simulink model "AllModeswithRA"  (R2022a)
settings: Solver=FixedStepAuto  StartTime=0.0  StopTime=10.0  FixedStep=1e-3  RelTol=1e-3  EnableMultiTasking=on
undefined symbols (not defined in the file): D0, D1, D10, D11, D12, D13, D2, D3, D4, D5, D6, D7, D8, D9, PTA0, PTA1, PTA2, PTB23, PTB9, PTC16, PTC17, PTC2, PTC3, PTC4, PTD0, PTD1, PTD2, PTD3
libraries: frdmk64flib x15, dspstat3 x1
settings Model: ExtModeTrigDuration=5  Creator=kemij  LastModifiedBy=kemij
settings OptimizationCC: EnhancedBackFolding=on  PassReuseOutputArgsAs=Individual arguments  ZeroExternalMemoryAtStartup=off  ZeroInternalMemoryAtStartup=off  MaxStackSize=64  OptimizeBlockOrder=speed  DifferentSizesBufferReuse=on  OptimizationCustomize=off  EfficientTunableParamExpr=on
settings DebuggingCC: ParameterTunabilityLossMsg=error
settings HardwareCC: ProdBitPerPointer=32  ProdBitPerSizeT=32  ProdBitPerPtrDiffT=32  ProdLargestAtomicInteger=Long  ProdLargestAtomicFloat=Double  ProdWordSize=32  ProdHWDeviceType=ARM Compatible->ARM Cortex
settings SFSimCC: MATLABDynamicMemAlloc=off
settings RTWCC: SystemTargetFile=ert.tlc  HardwareBoard=NXP FRDM-K64F  TLCOptions="-aInlineSetEventsForThisBaseRateFcn=TLC_FALSE -aSuppressMultiTaskScheduler=TLC_FALSE  -aRateBasedStepFcn=0"  TemplateMakefile=ert_default_tmf  Toolchain=GNU Tools for ARM Embedded Processors
settings CodeAppCC: ForceParamTrailComments=on  IgnoreCustomStorageClasses=off  OperatorAnnotations=on  SimulinkDataObjDesc=on  SFDataObjDesc=on  InsertBlockDesc=on
settings ERTTargetCC: ExtModeTransport=4  ExtModeMexFile=sendToCommService

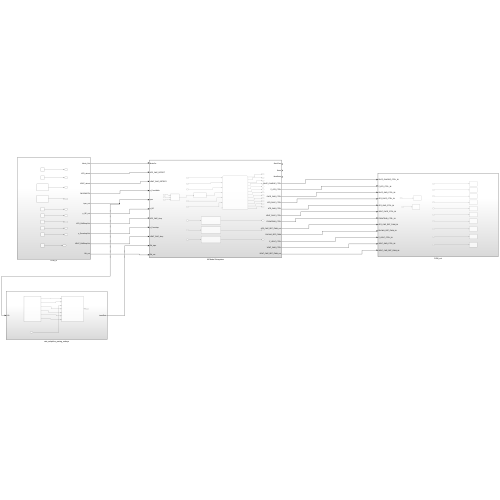
[thumbnail: Simulink's stored preview of the top-level diagram]
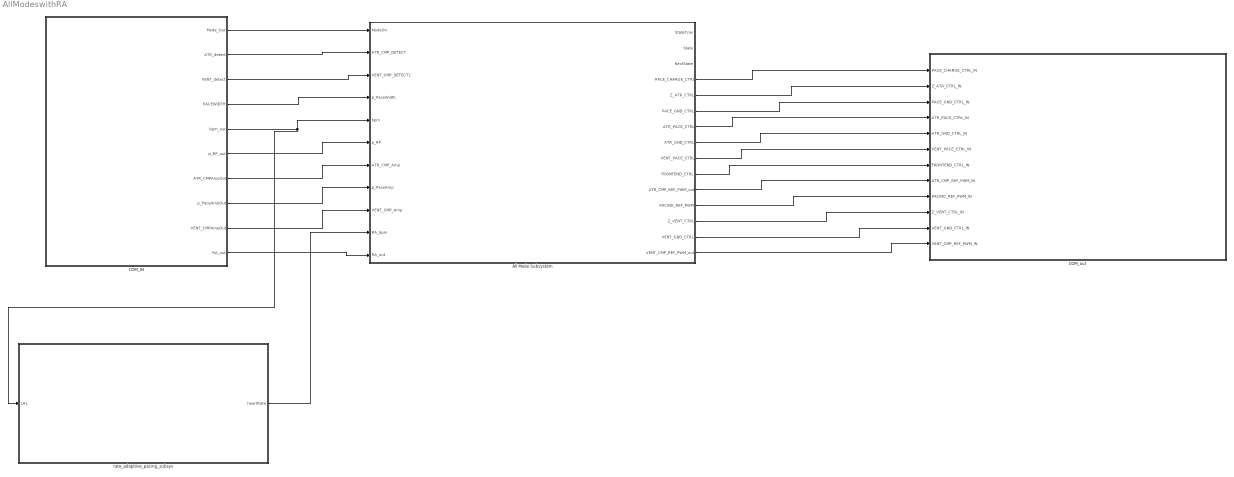
== system AllModeswithRA ==
  All Mode Subsystem : Subsystem
  COM_IN : Subsystem
  COM_out : Subsystem
  rate_adaptiive_pacing_subsys : Subsystem
  wires:
  COM_IN/3(VENT_detect) -> All Mode Subsystem/3(VENT_CMP_DETECT1)
  rate_adaptiive_pacing_subsys/1(heartRate) -> All Mode Subsystem/10(RA_bpm)
  COM_IN/10(RA_out) -> All Mode Subsystem/11(RA_out)
  COM_IN/2(ATR_detect) -> All Mode Subsystem/2(ATR_CMP_DETECT)
  All Mode Subsystem/13(Z_VENT_CTRL) -> COM_out/10(Z_VENT_CTRL_IN)
  All Mode Subsystem/15(VENT_CMP_REF_PWM_out) -> COM_out/12(VENT_CMP_REF_PWM_IN)
  COM_IN/6(p_RP_out) -> All Mode Subsystem/6(p_RP)
  COM_IN/1(Mode_Out) -> All Mode Subsystem/1(ModeOn)
  All Mode Subsystem/8(ATR_GND_CTRL) -> COM_out/5(ATR_GND_CTRL_IN)
  All Mode Subsystem/14(VENT_GND_CTRL) -> COM_out/11(VENT_GND_CTRL_IN)
  All Mode Subsystem/9(VENT_PACE_CTRL) -> COM_out/6(VENT_PACE_CTRL_IN)
  All Mode Subsystem/10(FRONTEND_CTRL) -> COM_out/7(FRONTEND_CTRL_IN)
  All Mode Subsystem/6(PACE_GND_CTRL) -> COM_out/3(PACE_GND_CTRL_IN)
  All Mode Subsystem/4(PACE_CHARGE_CTRL) -> COM_out/1(PACE_CHARGE_CTRL_IN)
  All Mode Subsystem/11(ATR_CMP_REF_PWM_out) -> COM_out/8(ATR_CMP_REF_PWM_IN)
  All Mode Subsystem/7(ATR_PACE_CTRL) -> COM_out/4(ATR_PACE_CTRL_IN)
  All Mode Subsystem/5(Z_ATR_CTRL) -> COM_out/2(Z_ATR_CTRL_IN)
  All Mode Subsystem/12(PACING_REF_PWM) -> COM_out/9(PACING_REF_PWM_IN)
  COM_IN/4(PACEWIDTH) -> All Mode Subsystem/4(p_PaceWidth)
  COM_IN/9(VENT_CMPAmpOut) -> All Mode Subsystem/9(VENT_CMP_Amp)
  COM_IN/5(bpm_out) -> rate_adaptiive_pacing_subsys/1(LRL), All Mode Subsystem/5(bpm)
  COM_IN/8(p_PaceAmpOut) -> All Mode Subsystem/8(p_PaceAmp)
  COM_IN/7(ATR_CMPAmpOut) -> All Mode Subsystem/7(ATR_CMP_Amp)

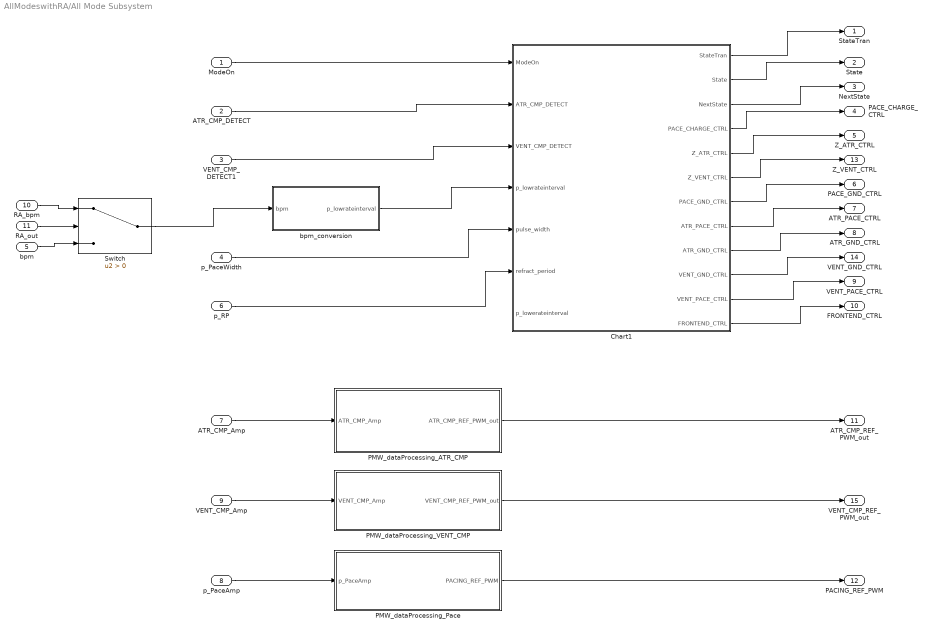
== system AllModeswithRA/All Mode Subsystem ==
  ModeOn : Inport
  ATR_CMP_DETECT : Inport  Port=2
  VENT_CMP_DETECT1 : Inport  Port=3
  p_PaceWidth : Inport  Port=4
  bpm : Inport  Port=5
  p_RP : Inport  Port=6
  ATR_CMP_Amp : Inport  Port=7
  p_PaceAmp : Inport  Port=8
  VENT_CMP_Amp : Inport  Port=9
  RA_bpm : Inport  Port=10
  RA_out : Inport  Port=11
  Chart1 : Stateflow chart  TreatAsAtomicUnit=on
      settings: PortSchema="{\"entries\":[{\"content\":{\"sides\":[{\"content\":{\"connectorIds\":[\"In1\",\"In2\",\"In3\",\"In4\",\"In5\",\"In6\",\"In7\"]},\"type\":\"ConnectorPlacement.EquallySpacedRectSide\",\"uuid\":\"7ea964f2-2529-4e69-b20d-c2fa6008c3a7\"},{\"content\":{\"connectorIds\":[\"Out12\",\"Out1\",\"Out11\",\"Out2\",\"Out3\",\"Out4\",\"Out5\",\"Out6\",\"Out7\",\"Out8\",\"Out9\",\"Out10\"],\"side\":\"RIGHT\"},\"type\":\"ConnectorPlacement.EquallySpacedRectSide\",\"uuid\":\"c561387b-bc02-43ab-893b-c9cb757a1c6a\"},{\"content\":{\"connectorIds\":[],\"side\":\"TOP\"},\"type\":\"ConnectorPlacement.EquallySpacedRectSide\",\"uuid\":\"1f667392-9a0f-4cad-82e3-6fe4d50b6af4\"}]},\"type\":\"ConnectorPlacement.EquallySpacedConnector\",\"uuid\":\"bd362c40-ffc0-452d-8626-3f1602423ca2\"}],\"packageUris\":[\"http://schema.mathworks.com/mf0/Connector/R2020b\"],\"version\":\"1.0\"}"
  PMW_dataProcessing_ATR_CMP : Subsystem
  PMW_dataProcessing_Pace : Subsystem
  PMW_dataProcessing_VENT_CMP : Subsystem
  Switch : Switch  Criteria=u2 > Threshold  SaturateOnIntegerOverflow=off  InputSameDT=off
  bpm_conversion : Subsystem
  StateTran : Outport
  State : Outport  Port=2
  NextState : Outport  Port=3
  PACE_CHARGE_CTRL : Outport  Port=4
  Z_ATR_CTRL : Outport  Port=5
  PACE_GND_CTRL : Outport  Port=6
  ATR_PACE_CTRL : Outport  Port=7
  ATR_GND_CTRL : Outport  Port=8
  VENT_PACE_CTRL : Outport  Port=9
  FRONTEND_CTRL : Outport  Port=10
  ATR_CMP_REF_PWM_out : Outport  Port=11
  PACING_REF_PWM : Outport  Port=12
  Z_VENT_CTRL : Outport  Port=13
  VENT_GND_CTRL : Outport  Port=14
  VENT_CMP_REF_PWM_out : Outport  Port=15
  wires:
  Chart1/10(FRONTEND_CTRL) -> FRONTEND_CTRL/1
  Chart1/9(VENT_PACE_CTRL) -> VENT_PACE_CTRL/1
  Chart1/7(ATR_GND_CTRL) -> ATR_GND_CTRL/1
  Chart1/6(ATR_PACE_CTRL) -> ATR_PACE_CTRL/1
  Chart1/5(PACE_GND_CTRL) -> PACE_GND_CTRL/1
  Chart1/3(Z_ATR_CTRL) -> Z_ATR_CTRL/1
  Chart1/2(PACE_CHARGE_CTRL) -> PACE_CHARGE_CTRL/1
  p_RP/1 -> Chart1/6(refract_period)
  p_PaceWidth/1 -> Chart1/5(pulse_width)
  ATR_CMP_DETECT/1 -> Chart1/2(ATR_CMP_DETECT)
  Chart1/1(State) -> State/1
  ModeOn/1 -> Chart1/1(ModeOn)
  Chart1/4(Z_VENT_CTRL) -> Z_VENT_CTRL/1
  Chart1/8(VENT_GND_CTRL) -> VENT_GND_CTRL/1
  VENT_CMP_DETECT1/1 -> Chart1/3(VENT_CMP_DETECT)
  ATR_CMP_Amp/1 -> PMW_dataProcessing_ATR_CMP/1(ATR_CMP_Amp)
  p_PaceAmp/1 -> PMW_dataProcessing_Pace/1(p_PaceAmp)
  VENT_CMP_Amp/1 -> PMW_dataProcessing_VENT_CMP/1(VENT_CMP_Amp)
  PMW_dataProcessing_Pace/1(PACING_REF_PWM) -> PACING_REF_PWM/1
  PMW_dataProcessing_VENT_CMP/1(VENT_CMP_REF_PWM_out) -> VENT_CMP_REF_PWM_out/1
  PMW_dataProcessing_ATR_CMP/1(ATR_CMP_REF_PWM_out) -> ATR_CMP_REF_PWM_out/1
  bpm_conversion/1(p_lowrateinterval) -> Chart1/4(p_lowrateinterval)
  Chart1/11(NextState) -> NextState/1
  Chart1/12(StateTran) -> StateTran/1
  RA_out/1 -> Switch/2
  RA_bpm/1 -> Switch/1
  bpm/1 -> Switch/3
  Switch/1 -> bpm_conversion/1(bpm)

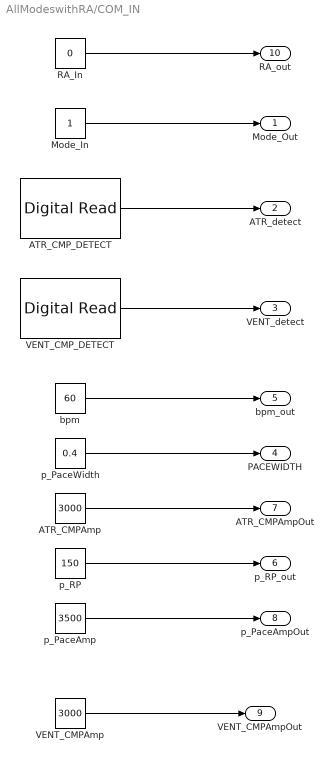
== system AllModeswithRA/COM_IN ==
  ATR_CMPAmp : Constant  Value=3000
  ATR_CMP_DETECT : frdmk64flib/Digital Read  Whichpin=PTC16 (D0)  SampleTime=-1
  Mode_In : Constant
  RA_In : Constant  Value=0
  VENT_CMPAmp : Constant  Value=3000
  VENT_CMP_DETECT : frdmk64flib/Digital Read  Whichpin=PTC17 (D1)  SampleTime=-1
  bpm : Constant  Value=60
  p_PaceAmp : Constant  Value=3500
  p_PaceWidth : Constant  Value=0.4
  p_RP : Constant  Value=150
  Mode_Out : Outport
  ATR_detect : Outport  Port=2
  VENT_detect : Outport  Port=3
  PACEWIDTH : Outport  Port=4
  bpm_out : Outport  Port=5
  p_RP_out : Outport  Port=6
  ATR_CMPAmpOut : Outport  Port=7
  p_PaceAmpOut : Outport  Port=8
  VENT_CMPAmpOut : Outport  Port=9
  RA_out : Outport  Port=10
  wires:
  Mode_In/1 -> Mode_Out/1
  ATR_CMP_DETECT/1 -> ATR_detect/1
  bpm/1 -> bpm_out/1
  ATR_CMPAmp/1 -> ATR_CMPAmpOut/1
  VENT_CMP_DETECT/1 -> VENT_detect/1
  p_PaceWidth/1 -> PACEWIDTH/1
  p_RP/1 -> p_RP_out/1
  p_PaceAmp/1 -> p_PaceAmpOut/1
  VENT_CMPAmp/1 -> VENT_CMPAmpOut/1
  RA_In/1 -> RA_out/1

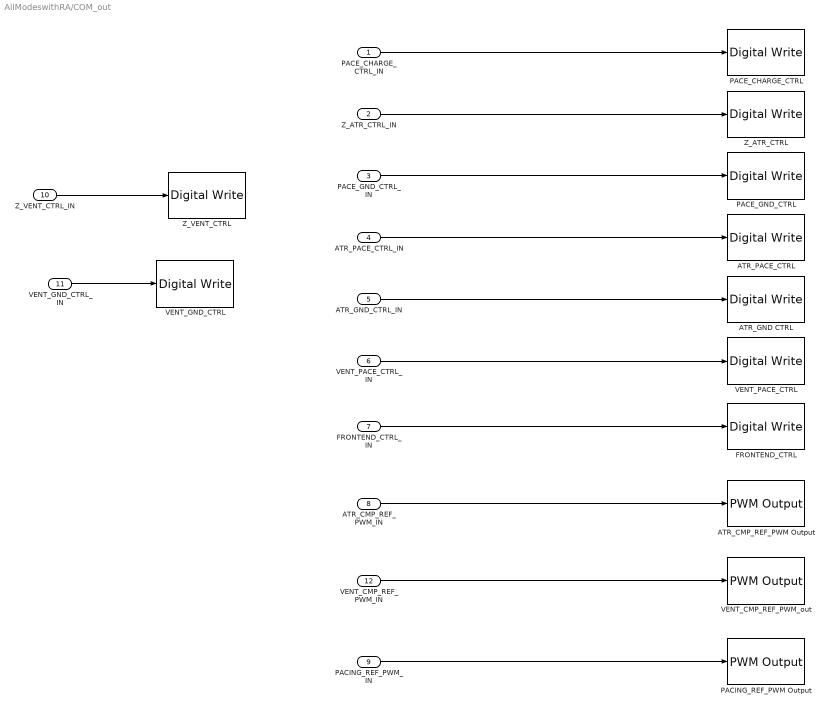
== system AllModeswithRA/COM_out ==
  PACE_CHARGE_CTRL_IN : Inport
  Z_ATR_CTRL_IN : Inport  Port=2
  PACE_GND_CTRL_IN : Inport  Port=3
  ATR_PACE_CTRL_IN : Inport  Port=4
  ATR_GND_CTRL_IN : Inport  Port=5
  VENT_PACE_CTRL_IN : Inport  Port=6
  FRONTEND_CTRL_IN : Inport  Port=7
  ATR_CMP_REF_PWM_IN : Inport  Port=8
  PACING_REF_PWM_IN : Inport  Port=9
  Z_VENT_CTRL_IN : Inport  Port=10
  VENT_GND_CTRL_IN : Inport  Port=11
  VENT_CMP_REF_PWM_IN : Inport  Port=12
  ATR_CMP_REF_PWM Output : frdmk64flib/PWM Output  Whichpin=PTC2 (D6)  InitialFrequency=2000  InitialDutyCycle=0
  ATR_GND CTRL : frdmk64flib/Digital Write  Whichpin=PTD2 (D11)
  ATR_PACE_CTRL : frdmk64flib/Digital Write  Whichpin=PTA0 (D8)
  FRONTEND_CTRL : frdmk64flib/Digital Write  Whichpin=PTD1 (D13)
  PACE_CHARGE_CTRL : frdmk64flib/Digital Write  Whichpin=PTB9 (D2)
  PACE_GND_CTRL : frdmk64flib/Digital Write  Whichpin=PTD0 (D10)
  PACING_REF_PWM Output : frdmk64flib/PWM Output  Whichpin=PTA2 (D5)  InitialFrequency=2000  InitialDutyCycle=0
  VENT_CMP_REF_PWM_out : frdmk64flib/PWM Output  Whichpin=PTA1 (D3)  InitialFrequency=2000  InitialDutyCycle=0
  VENT_GND_CTRL : frdmk64flib/Digital Write  Whichpin=PTD3 (D12)
  VENT_PACE_CTRL : frdmk64flib/Digital Write  Whichpin=PTC4 (D9)
  Z_ATR_CTRL : frdmk64flib/Digital Write  Whichpin=PTB23 (D4)
  Z_VENT_CTRL : frdmk64flib/Digital Write  Whichpin=PTC3 (D7)
  wires:
  PACE_CHARGE_CTRL_IN/1 -> PACE_CHARGE_CTRL/1
  PACE_GND_CTRL_IN/1 -> PACE_GND_CTRL/1
  Z_ATR_CTRL_IN/1 -> Z_ATR_CTRL/1
  ATR_PACE_CTRL_IN/1 -> ATR_PACE_CTRL/1
  ATR_GND_CTRL_IN/1 -> ATR_GND CTRL/1
  VENT_PACE_CTRL_IN/1 -> VENT_PACE_CTRL/1
  FRONTEND_CTRL_IN/1 -> FRONTEND_CTRL/1
  PACING_REF_PWM_IN/1 -> PACING_REF_PWM Output/1
  ATR_CMP_REF_PWM_IN/1 -> ATR_CMP_REF_PWM Output/1
  VENT_GND_CTRL_IN/1 -> VENT_GND_CTRL/1
  Z_VENT_CTRL_IN/1 -> Z_VENT_CTRL/1
  VENT_CMP_REF_PWM_IN/1 -> VENT_CMP_REF_PWM_out/1

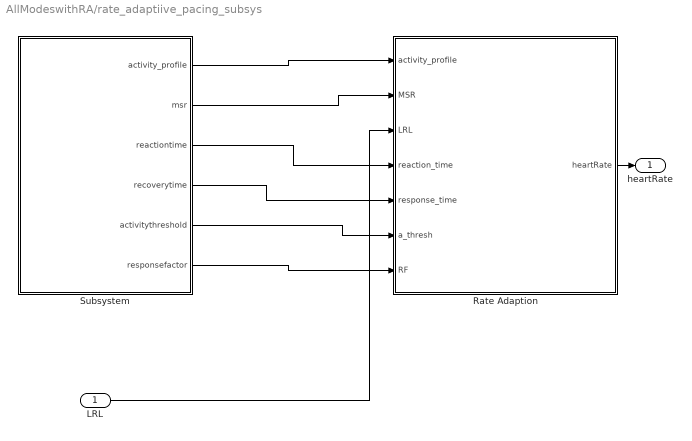
== system AllModeswithRA/rate_adaptiive_pacing_subsys ==
  LRL : Inport
  Rate Adaption : Subsystem
  Subsystem : Subsystem
  heartRate : Outport
  wires:
  Rate Adaption/1(heartRate) -> heartRate/1
  Subsystem/1(activity_profile) -> Rate Adaption/1(activity_profile)
  Subsystem/3(reactiontime) -> Rate Adaption/4(reaction_time)
  Subsystem/4(recoverytime) -> Rate Adaption/5(response_time)
  Subsystem/5(activitythreshold) -> Rate Adaption/6(a_thresh)
  Subsystem/6(responsefactor) -> Rate Adaption/7(RF)
  Subsystem/2(msr) -> Rate Adaption/2(MSR)
  LRL/1 -> Rate Adaption/3(LRL)

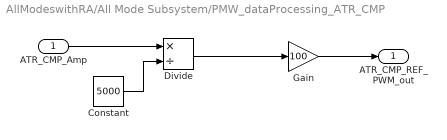
== system AllModeswithRA/All Mode Subsystem/PMW_dataProcessing_ATR_CMP ==
  ATR_CMP_Amp : Inport
  Constant : Constant  Value=5000
  Divide : Product  Inputs=*/
  Gain : Gain  Gain=100
  ATR_CMP_REF_PWM_out : Outport
  wires:
  Divide/1 -> Gain/1
  Constant/1 -> Divide/2
  ATR_CMP_Amp/1 -> Divide/1
  Gain/1 -> ATR_CMP_REF_PWM_out/1

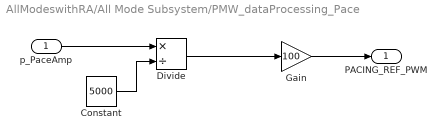
== system AllModeswithRA/All Mode Subsystem/PMW_dataProcessing_Pace ==
  p_PaceAmp : Inport
  Constant : Constant  Value=5000
  Divide : Product  Inputs=*/
  Gain : Gain  Gain=100
  PACING_REF_PWM : Outport
  wires:
  Divide/1 -> Gain/1
  Constant/1 -> Divide/2
  p_PaceAmp/1 -> Divide/1
  Gain/1 -> PACING_REF_PWM/1

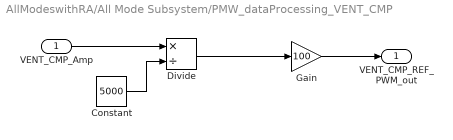
== system AllModeswithRA/All Mode Subsystem/PMW_dataProcessing_VENT_CMP ==
  VENT_CMP_Amp : Inport
  Constant : Constant  Value=5000
  Divide : Product  Inputs=*/
  Gain : Gain  Gain=100
  VENT_CMP_REF_PWM_out : Outport
  wires:
  Divide/1 -> Gain/1
  Constant/1 -> Divide/2
  VENT_CMP_Amp/1 -> Divide/1
  Gain/1 -> VENT_CMP_REF_PWM_out/1

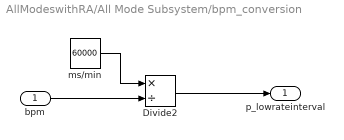
== system AllModeswithRA/All Mode Subsystem/bpm_conversion ==
  bpm : Inport
  Divide2 : Product  Inputs=*/
  ms/min : Constant  Value=60000
  p_lowrateinterval : Outport
  wires:
  ms/min/1 -> Divide2/1
  bpm/1 -> Divide2/2
  Divide2/1 -> p_lowrateinterval/1

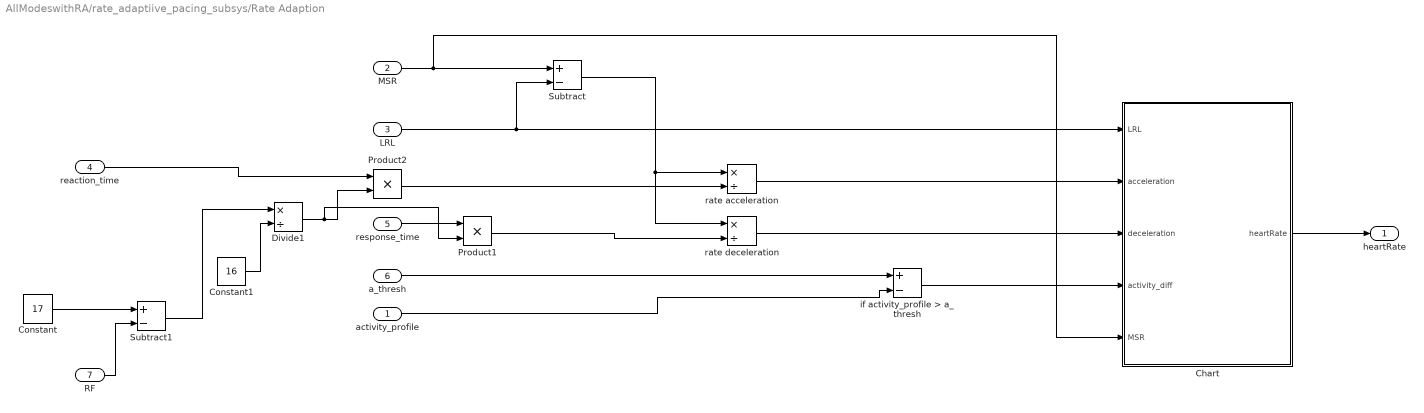
== system AllModeswithRA/rate_adaptiive_pacing_subsys/Rate Adaption ==
  activity_profile : Inport
  MSR : Inport  Port=2
  LRL : Inport  Port=3
  reaction_time : Inport  Port=4
  response_time : Inport  Port=5
  a_thresh : Inport  Port=6
  RF : Inport  Port=7
  Chart : Stateflow chart  TreatAsAtomicUnit=on
      settings: PortSchema="{\"entries\":[{\"content\":{\"sides\":[{\"content\":{\"connectorIds\":[\"In5\",\"In1\",\"In3\",\"In2\",\"In4\"]},\"type\":\"ConnectorPlacement.EquallySpacedRectSide\",\"uuid\":\"f1bfb65c-a3e0-488b-a51c-ed381b80a0d3\"},{\"content\":{\"connectorIds\":[\"Out1\"],\"side\":\"RIGHT\"},\"type\":\"ConnectorPlacement.EquallySpacedRectSide\",\"uuid\":\"38293472-2491-4ffe-ba83-6a5f72f7d4c8\"},{\"content\":{\"connectorIds\":[],\"side\":\"TOP\"},\"type\":\"ConnectorPlacement.EquallySpacedRectSide\",\"uuid\":\"d4d219f0-2dab-436b-b9c2-781e051d4797\"}]},\"type\":\"ConnectorPlacement.EquallySpacedConnector\",\"uuid\":\"faf9de58-f900-4f39-b014-8d2778c5d5cd\"}],\"packageUris\":[\"http://schema.mathworks.com/mf0/Connector/R2020b\"],\"version\":\"1.0\"}"
  Constant : Constant  Value=17
  Constant1 : Constant  Value=16
  Divide1 : Product  Inputs=*/
  Product1 : Product
  Product2 : Product
  Subtract : Sum  Inputs=+-
  Subtract1 : Sum  Inputs=+-
  if activity_profile > a_thresh : Sum  Inputs=+-
  rate acceleration : Product  Inputs=*/
  rate deceleration : Product  Inputs=*/
  heartRate : Outport
  wires:
  MSR/1 -> Chart/4(MSR), Subtract/1
  Chart/1(heartRate) -> heartRate/1
  LRL/1 -> Chart/5(LRL), Subtract/2
  Subtract/1 -> rate deceleration/1, rate acceleration/1
  RF/1 -> Subtract1/2
  rate acceleration/1 -> Chart/1(acceleration)
  rate deceleration/1 -> Chart/3(deceleration)
  if activity_profile > a_thresh/1 -> Chart/2(activity_diff)
  a_thresh/1 -> if activity_profile > a_thresh/1
  activity_profile/1 -> if activity_profile > a_thresh/2
  Product2/1 -> rate acceleration/2
  Constant/1 -> Subtract1/1
  Subtract1/1 -> Divide1/1
  Constant1/1 -> Divide1/2
  reaction_time/1 -> Product2/1
  Divide1/1 -> Product2/2, Product1/2
  response_time/1 -> Product1/1
  Product1/1 -> rate deceleration/2

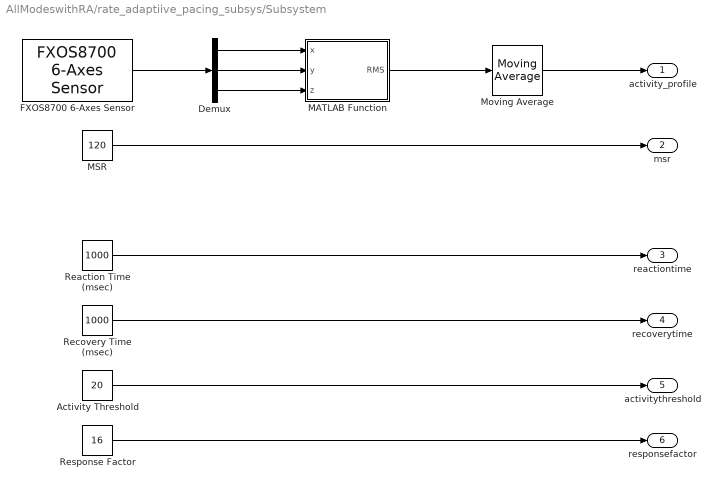
== system AllModeswithRA/rate_adaptiive_pacing_subsys/Subsystem ==
  Activity Threshold : Constant  Value=20
  Demux : Demux  Outputs=3
  FXOS8700 6-Axes Sensor : frdmk64flib/FXOS8700 6-Axes Sensor  Activesensor=Accelerometer only  ODR=800Hz  HybridODR=400Hz  Accelfullrange=-4g to +4g  SampleTime=-1
  MATLAB Function : MATLAB Function  TreatAsAtomicUnit=on
  MSR : Constant  Value=120
  Moving Average : dspstat3/Moving Average  Method=Sliding window  ForgettingFactorPort=off  SpecifyWindowLength=on  WindowLength=4  ForgettingFactor=0.9  SimulateUsing=Code generation
  Reaction Time (msec) : Constant  Value=1000
  Recovery Time (msec) : Constant  Value=1000
  Response Factor : Constant  Value=16
  activity_profile : Outport
  msr : Outport  Port=2
  reactiontime : Outport  Port=3
  recoverytime : Outport  Port=4
  activitythreshold : Outport  Port=5
  responsefactor : Outport  Port=6
  wires:
  Moving Average/1 -> activity_profile/1
  MSR/1 -> msr/1
  Reaction Time (msec)/1 -> reactiontime/1
  Recovery Time (msec)/1 -> recoverytime/1
  Activity Threshold/1 -> activitythreshold/1
  Response Factor/1 -> responsefactor/1
  Demux/3 -> MATLAB Function/3(z)
  Demux/2 -> MATLAB Function/2(y)
  MATLAB Function/1(RMS) -> Moving Average/1
  Demux/1 -> MATLAB Function/1(x)
  FXOS8700 6-Axes Sensor/1 -> Demux/1

== matlab function AllModeswithRA/rate_adaptiive_pacing_subsys/Subsystem/MATLAB Function ==
  data: x input; RMS output; y input; z input
function RMS = calc_RMS(x,y,z)

RMS = sqrt((x^2 + y^2 + z^2)/3.0);

== stateflow chart AllModeswithRA/All Mode Subsystem/Chart1 ==
  state AOO_Charging_Discharging
    entry:
    StateTran = false
    NextState = 0
    ATR_PACE_CTRL = false
    VENT_PACE_CTRL=false
    PACE_CHARGE_CTRL = true
    ATR_GND_CTRL = true
    PACE_GND_CTRL = true
    Z_ATR_CTRL=false
    State = 1
    exit:
    StateTran = true
  state AOO_Pace_Heart
    entry:
    StateTran = false
    NextState = 0
    ATR_PACE_CTRL = true
    PACE_CHARGE_CTRL = false
    PACE_GND_CTRL = true
    ATR_GND_CTRL = false
    State = 2
    exit:
    StateTran = true
  state VOO_VENT_Charging_Discharging
    entry:
    NextState = 0
    VENT_PACE_CTRL = false
    ATR_PACE_CTRL = false
    PACE_CHARGE_CTRL = true
    VENT_GND_CTRL = true
    PACE_GND_CTRL = true
    Z_VENT_CTRL=false
    State = 3
    StateTran = false
    exit:
    StateTran = true
  state VOO_VENT_Pace_Heart
    entry:
    NextState = 0
    StateTran = false
    VENT_PACE_CTRL = true
    PACE_CHARGE_CTRL = false
    PACE_GND_CTRL = true
    VENT_GND_CTRL = false
    State = 4
    exit:
    StateTran = true
  state AAI_Pulse_Sensed
    entry:
    NextState = 0
    %FRONTEND_CTRL=false
    State = 6
    StateTran = false
    exit:
    StateTran = true
    wait_time=refract_period
  state StateOff
    %This state tells the pacemaker which
    %mode it should run, which is decided
    %by ModeOn and is checked on the
    %transistion conditions.
    entry:
    %Initialize all states to 0 or false, since
    %the pacemaker should do nothing in this
    %state.
    StateTran = false
    State = 0
    NextState = 0
    PACE_CHARGE_CTRL = false
    Z_ATR_CTRL = false
    Z_VENT_CTRL = false
    PACE_GND_CTRL = false
    ATR_PACE_CTRL = false
    ATR_GND_CTRL = false
    VENT_GND_CTRL = false
    VENT_PACE_CTRL = false
    FRONTEND_CTRL = false
    exit:
    StateTran = true
    wait_time=pulse_width
  state AAI_Charging_Discharging
    entry:
    NextState = 0
    ATR_PACE_CTRL = false
    VENT_PACE_CTRL=false
    PACE_CHARGE_CTRL = true
    ATR_GND_CTRL = true
    PACE_GND_CTRL = true
    Z_ATR_CTRL=false
    FRONTEND_CTRL=true
    State = 5
    StateTran = false
    exit:
    StateTran = true
  state AAI_Pace_Heart
    entry:
    NextState = 0
    ATR_PACE_CTRL = true
    PACE_CHARGE_CTRL = false
    PACE_GND_CTRL = true
    ATR_GND_CTRL = false
    State = 7
    StateTran = false
    exit:
    StateTran = true
    wait_time=pulse_width
  state VVI_Pulse_Sensed
    entry:
    NextState = 0
    %FRONTEND_CTRL=false
    State = 9
    StateTran = false
    exit:
    StateTran = true
    wait_time=refract_period
  state VVI_Charging_Discharging
    entry:
    NextState = 0
    ATR_PACE_CTRL = false
    VENT_PACE_CTRL=false
    PACE_CHARGE_CTRL = true
    VENT_GND_CTRL = true
    PACE_GND_CTRL = true
    Z_VENT_CTRL=false
    FRONTEND_CTRL=true
    State = 8
    StateTran = false
    exit:
    StateTran = true
  state VVI_Pace_Heart
    entry:
    NextState = 0
    VENT_PACE_CTRL = true
    PACE_CHARGE_CTRL = false
    PACE_GND_CTRL = true
    VENT_GND_CTRL = false
    State = 10
    StateTran = false
    exit:
    StateTran = true
    wait_time=pulse_width
  AOO_Charging_Discharging -> AOO_Pace_Heart : after(p_lowrateinterval-pulse_width,msec) / {NextState = 2}
  StateOff -> AOO_Charging_Discharging [order 4] : [ModeOn==1] / {NextState = 1}
  AOO_Pace_Heart -> AOO_Charging_Discharging : after(pulse_width,msec) / {NextState = 1}
  VOO_VENT_Charging_Discharging -> VOO_VENT_Pace_Heart : after(p_lowerateinterval-pulse_width,msec) / {NextState = 4}
  VOO_VENT_Pace_Heart -> VOO_VENT_Charging_Discharging : after(pulse_width,msec) / {NextState = 3}
  StateOff -> VOO_VENT_Charging_Discharging [order 3] : [ModeOn==2] / {NextState = 3}
  (default) -> StateOff
  AAI_Pulse_Sensed -> AAI_Charging_Discharging : [after(refract_period,msec)] / {NextState = 5}
  AAI_Charging_Discharging -> AAI_Pulse_Sensed [order 2] : [ATR_CMP_DETECT == 1] / {NextState = 6}
  StateOff -> AAI_Charging_Discharging [order 1] : [ModeOn==3] / {NextState = 5}
  AAI_Charging_Discharging -> AAI_Pace_Heart [order 1] : [after(p_lowrateinterval-wait_time,msec)] / {NextState = 7}
  AAI_Pace_Heart -> AAI_Charging_Discharging : after(pulse_width,msec) / {NextState = 5}
  StateOff -> VVI_Charging_Discharging [order 2] : [ModeOn==4] / {NextState = 8}
  VVI_Pulse_Sensed -> VVI_Charging_Discharging : [after(refract_period,msec)] / {NextState = 8}
  VVI_Charging_Discharging -> VVI_Pulse_Sensed [order 2] : [VENT_CMP_DETECT == 1] / {NextState = 9}
  VVI_Charging_Discharging -> VVI_Pace_Heart [order 1] : [after(p_lowrateinterval-wait_time,msec)] / {NextState = 10}
  VVI_Pace_Heart -> VVI_Charging_Discharging : after(pulse_width,msec) / {NextState = 8}
  data: ModeOn input; State output int8; ATR_CMP_DETECT input boolean; VENT_CMP_DETECT input; p_lowrateinterval input; PACE_CHARGE_CTRL output boolean; Z_ATR_CTRL output boolean; Z_VENT_CTRL output boolean; PACE_GND_CTRL output boolean; ATR_PACE_CTRL output boolean; ATR_GND_CTRL output boolean; VENT_GND_CTRL output boolean; pulse_width input; VENT_PACE_CTRL output boolean; refract_period input; FRONTEND_CTRL output boolean; NextState output int8; StateTran output boolean; wait_time local; p_lowerateinterval input

== stateflow chart AllModeswithRA/rate_adaptiive_pacing_subsys/Rate Adaption/Chart ==
  state IncreaseHeartRate
    during:
    activity_time = elapsed(msec)
    heartRate = heartRate + acceleration*activity_time
  state HOLDSensorRate
    during:
    heartRate = MSR
  state IDLE
    entry:
    heartRate = LRL
    activity_time = 0
    zero_activity_time = 0
  state ActivitySensed
    %activity has been sensed
  state HOLDLRL
    during:
    heartRate = LRL
  state DecreaseHeartRate
    % decrease rate until there is zero activity (0 bpm)
    during:
    zero_activity_time = elapsed(msec)
    heartRate = heartRate - deceleration*zero_activity_time
  (junction 15) -> IncreaseHeartRate [order 1] : [heartRate + acceleration*activity_time <MSR]
  IncreaseHeartRate -> (junction 26) : [heartRate==MSR || activity_diff<=0 ]
  ActivitySensed -> (junction 15) [order 2] : [activity_diff > 0]
  (junction 15) -> HOLDSensorRate [order 2] : [heartRate + acceleration*activity_time >= MSR]
  HOLDSensorRate -> (junction 26) : [activity_diff<=0]
  (default) -> IDLE
  IDLE -> ActivitySensed
  (junction 26) -> ActivitySensed
  HOLDLRL -> (junction 26) : [activity_diff>0]
  DecreaseHeartRate -> (junction 26) : [activity_diff>0||heartRate==LRL]
  ActivitySensed -> (junction 16) [order 1] : [activity_diff <= 0]
  (junction 16) -> HOLDLRL [order 2] : [heartRate - deceleration*zero_activity_time <= LRL]
  (junction 16) -> DecreaseHeartRate [order 1] : [heartRate - deceleration*zero_activity_time > LRL]
  data: acceleration input; activity_diff input; deceleration input; MSR input; activity_time local; LRL input; zero_activity_time local; heartRate output
